simulink model "RLC"  (Simulink 8.5)
settings: Solver=ode3  StartTime=0  StopTime=0.005  FixedStep=0.00001  RelTol=1e-3
settings Model: Creator=ASUS  LastModifiedBy=ASUS
settings DataIOCC: SignalLoggingSaveFormat=Dataset
settings OptimizationCC: ExpressionDepthLimit=128
settings DebuggingCC: UnderspecifiedInitializationDetection=Simplified  MergeDetectMultiDrivingBlocksExec=error  FcnCallInpInsideContextMsg=EnableAllAsError  StateNameClashWarn=none
settings GRTTargetCC: CombineOutputUpdateFcns=on  GRTInterface=off

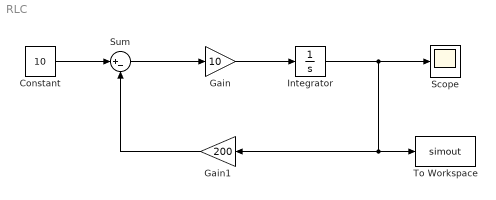
== system RLC ==
  Constant : Constant  Value=10
  Gain : Gain  Gain=10
  Gain1 : Gain  Gain=200
  Integrator : Integrator
  Scope : Scope
      settings: TimeRange=0.005
  Sum : Sum  Inputs=|+-
  To Workspace : ToWorkspace  VariableName=simout  SampleTime=-1
  wires:
  Constant/1 -> Sum/1
  Sum/1 -> Gain/1
  Integrator/1 -> To Workspace/1, Gain1/1, Scope/1
  Gain1/1 -> Sum/2
  Gain/1 -> Integrator/1
